simulink model "loopshaping_model"  (R2015a)
settings: Solver=ode45  StartTime=0.0  StopTime=10.0  RelTol=1e-3
values from neighbouring files (symbols this model uses):
  Cl = 8    [controller_parameters.m]
  gain = -0.03    [controller_parameters.m]
  Ke = -1.0000e+05    (= -100000)    [controller_parameters.m]
  Kl = 162    [controller_parameters.m]
  L = 0.0220    (= 0.022)    [controller_parameters.m]
  M = 1.35    [controller_parameters.m]
  pole1 = -100    [controller_parameters.m]
  R = 1.3    [controller_parameters.m]
  zero1 = -2.5+10i    [controller_parameters.m]
  zero2 = -2.5-10i    [controller_parameters.m]
settings Model: CovModelRefEnable=off  Creator=gsavaia  LastModifiedBy=GSavaia
settings DataIOCC: SaveFormat=Dataset
settings HardwareCC: ProdBitPerPointer=64  ProdLargestAtomicFloat=Float  ProdIntDivRoundTo=Zero  ProdEndianess=LittleEndian  ProdHWDeviceType=Specified
settings GRTTargetCC: GeneratePreprocessorConditionals=Use local settings

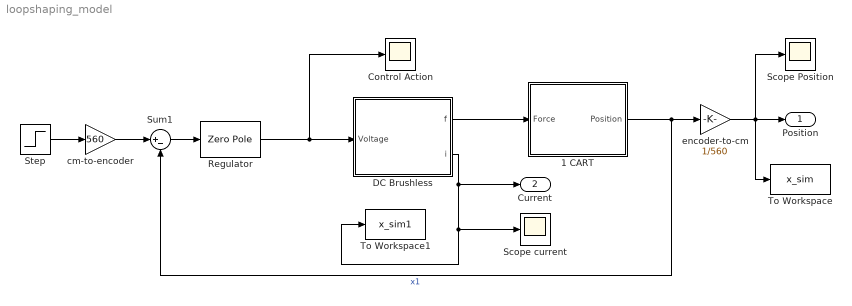
== system loopshaping_model ==
  1 CART : Subsystem
  Control Action : Scope
      settings: TimeRange=10  YMin=0  YMax=1000  SaveName=ScopeData4
  DC Brushless : Subsystem
  Regulator : ZeroPole  Zeros=[zero1, zero2]  Poles=[0, pole1]  Gain=gain
  Scope Position : Scope
      settings: YMin=-0.25393  YMax=2.28535
  Scope current : Scope
      settings: YMin=-0.525  YMax=4.725
  Step : Step  SampleTime=0
  Sum1 : Sum  Inputs=|+-
  To Workspace : ToWorkspace  VariableName=x_sim  SampleTime=-1
  To Workspace1 : ToWorkspace  VariableName=x_sim1  SampleTime=-1
  cm-to-encoder : Gain  Gain=560
  encoder-to-cm : Gain  Gain=1/560
  Position : Outport
  Current : Outport  Port=2
  wires:
  DC Brushless/1("f ") -> 1 CART/1(Force)
  1 CART/1(Position) -> encoder-to-cm/1, Sum1/2  "x1"
  Regulator/1 -> DC Brushless/1("Voltage "), Control Action/1
  DC Brushless/2(i) -> Current/1, To Workspace1/1, Scope current/1
  Sum1/1 -> Regulator/1
  cm-to-encoder/1 -> Sum1/1
  Step/1 -> cm-to-encoder/1
  encoder-to-cm/1 -> To Workspace/1, Position/1, Scope Position/1

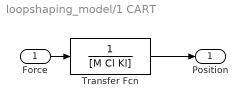
== system loopshaping_model/1 CART ==
  Force : Inport
  Transfer Fcn : TransferFcn  Denominator=[M Cl Kl]
  Position : Outport
  wires:
  Force/1 -> Transfer Fcn/1
  Transfer Fcn/1 -> Position/1

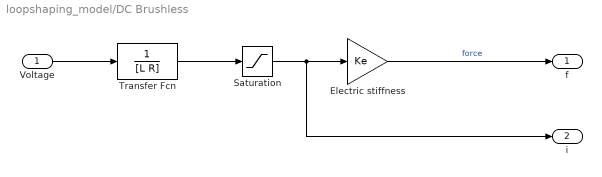
== system loopshaping_model/DC Brushless ==
  "Voltage " : Inport
  Electric stiffness : Gain  Gain=Ke
  Saturation : Saturate  UpperLimit=4.2  LowerLimit=-10
  Transfer Fcn : TransferFcn  Denominator=[L R]
  "f " : Outport
  i : Outport  Port=2
  wires:
  "Voltage "/1 -> Transfer Fcn/1
  Electric stiffness/1 -> "f "/1  "force"
  Transfer Fcn/1 -> Saturation/1
  Saturation/1 -> i/1, Electric stiffness/1
